simulink model "ex11"  (Simulink 8.7)
settings: Solver=FixedStepAuto  StartTime=0.0  StopTime=60  FixedStep=0.001  RelTol=1e-3
settings Model: Creator=Dinis  LastModifiedBy=Dinis
settings DataIOCC: LimitDataPoints=off  SaveFormat=Dataset
settings DebuggingCC: UnderspecifiedInitializationDetection=Simplified  MergeDetectMultiDrivingBlocksExec=error  ParameterOverflowMsg=none
settings HardwareCC: ProdBitPerPointer=64  ProdLargestAtomicFloat=Float  ProdIntDivRoundTo=Zero  ProdEndianess=LittleEndian  ProdWordSize=64  ProdHWDeviceType=Intel->x86-64 (Windows64)
settings ModelReferenceCC: PropagateSignalLabelsOutOfModel=on
settings ConfigComp: CovModelRefEnable=off

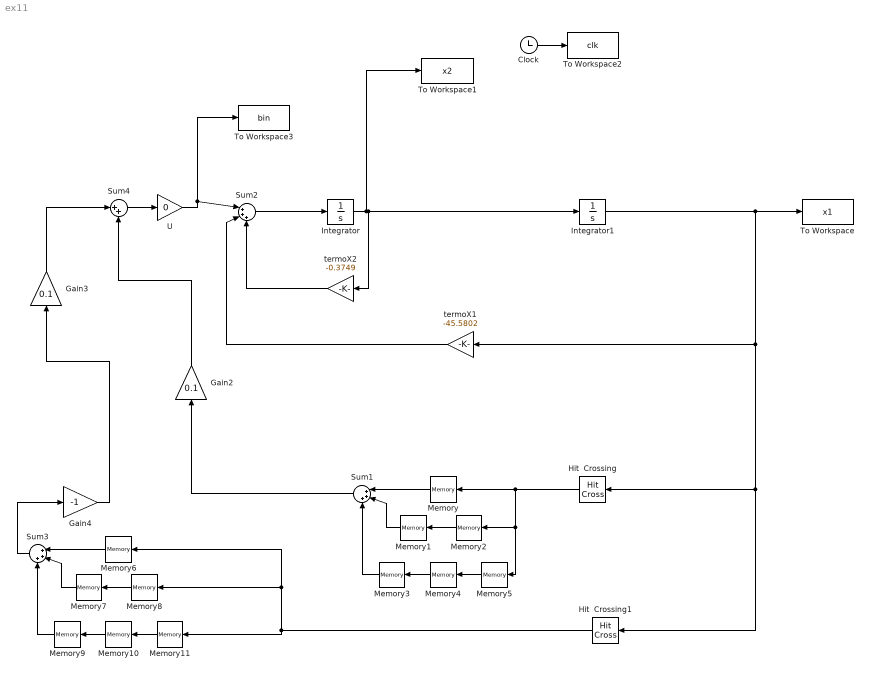
== system ex11 ==
  Clock : Clock
  Gain2 : Gain  Gain=0.1
  Gain3 : Gain  Gain=0.1
  Gain4 : Gain  Gain=-1
  Hit  Crossing : HitCross  HitCrossingDirection=rising
  Hit  Crossing1 : HitCross  HitCrossingDirection=falling
  Integrator : Integrator
  Integrator1 : Integrator  InitialCondition=pi/4
  Memory{,1..11} (12 alike) : Memory
  Sum1 : Sum  Inputs=|+++
  Sum2 : Sum  Inputs=|+++
  Sum3 : Sum  Inputs=|+++
  Sum4 : Sum  Inputs=|++
  To Workspace : ToWorkspace  VariableName=x1  SampleTime=-1
  To Workspace1 : ToWorkspace  VariableName=x2  SampleTime=-1
  To Workspace2 : ToWorkspace  VariableName=clk  SampleTime=-1
  To Workspace3 : ToWorkspace  VariableName=bin  SampleTime=-1
  U : Gain  Gain=0
  termoX1 : Gain  Gain=-45.5802
  termoX2 : Gain  Gain=-0.3749
  wires:
  Integrator1/1 -> To Workspace/1, Hit  Crossing1/1, Hit  Crossing/1, termoX1/1
  termoX1/1 -> Sum2/2
  Sum2/1 -> Integrator/1
  termoX2/1 -> Sum2/3
  Integrator/1 -> Integrator1/1, termoX2/1, To Workspace1/1
  U/1 -> To Workspace3/1, Sum2/1
  Clock/1 -> To Workspace2/1
  Hit  Crossing/1 -> Memory/1, Memory2/1, Memory5/1
  Memory/1 -> Sum1/1
  Sum1/1 -> Gain2/1
  Memory2/1 -> Memory1/1
  Memory1/1 -> Sum1/2
  Memory4/1 -> Memory3/1
  Memory5/1 -> Memory4/1
  Memory3/1 -> Sum1/3
  Hit  Crossing1/1 -> Memory11/1, Memory6/1, Memory8/1
  Memory6/1 -> Sum3/1
  Memory8/1 -> Memory7/1
  Memory7/1 -> Sum3/2
  Memory10/1 -> Memory9/1
  Memory11/1 -> Memory10/1
  Memory9/1 -> Sum3/3
  Sum3/1 -> Gain4/1
  Gain4/1 -> Gain3/1
  Gain2/1 -> Sum4/2
  Gain3/1 -> Sum4/1
  Sum4/1 -> U/1
